simulink model "DC_Motor_Control_PM"  (R2022b)
settings: Solver=ode23s  StartTime=0.0  StopTime=0.2  RelTol=1e-3  EnableMultiTasking=on
values from neighbouring files (symbols this model uses):
  B = 0.01    [PI_design_DC_PM.m]
  J = 6e-5    (= 6e-05)    [PI_design_DC_PM.m]
  K = Ke    (= 0.04)    [PI_design_DC_PM.m]
  kb_curr = 1/tauGc    (= 300)    [PI_design_DC_PM.m]
  kb_speed = 1/tauGm    (= 166.666666667)    [PI_design_DC_PM.m]
  ki_curr = Ccurr.Ki    [PI_design_DC_PM.m]
  ki_speed = Cspeed.Ki    [PI_design_DC_PM.m]
  kp_curr = Ccurr.Kp    [PI_design_DC_PM.m]
  kp_speed = Cspeed.Kp    [PI_design_DC_PM.m]
  La = 0.002    [PI_design_DC_PM.m]
  Ra = 0.6    [PI_design_DC_PM.m]
libraries: slpidlib x2
settings Model: Creator=matti  LastModifiedBy=benve
settings SolverCC: AlgebraicLoopSolver=TrustRegion
settings DataIOCC: LimitDataPoints=on  SaveFormat=Array  ReturnWorkspaceOutputs=off
settings OptimizationCC: LifeSpan=inf
settings DebuggingCC: SolverPrmCheckMsg=warning  UnconnectedInputMsg=warning  UnconnectedOutputMsg=warning  UnconnectedLineMsg=warning  SFUnexpectedBacktrackingDiag=warning  SFNoUnconditionalDefaultTransitionDiag=warning  SFExecutionAtInitializationDiag=none  SFMachineParentedDataDiag=warning  ArithmeticOperatorsInVariantConditions=warning
settings HardwareCC: ProdBitPerPointer=32  ProdBitPerSizeT=32  ProdBitPerPtrDiffT=32  ProdLargestAtomicFloat=None  ProdIntDivRoundTo=Undefined  ProdEndianess=Unspecified  ProdWordSize=32  ProdHWDeviceType=32-bit Generic
settings ModelReferenceCC: EnableRefExpFcnMdlSchedulingChecks=on  PropagateSignalLabelsOutOfModel=off
settings SFSimCC: SimUseLocalCustomCode=off  CustomCodeUndefinedFunction=UseInterfaceOnly
settings RTWCC: RTWUseLocalCustomCode=off
settings CodeAppCC: StateflowObjectComments=on
settings GRTTargetCC: TargetLangStandard=C89/C90 (ANSI)
settings ConfigComp: CovMetricSettings=dw  CovSaveCumulativeToWorkspaceVar=on  CovSaveSingleToWorkspaceVar=on  CovExternalEMLEnable=off  CovSFcnEnable=off

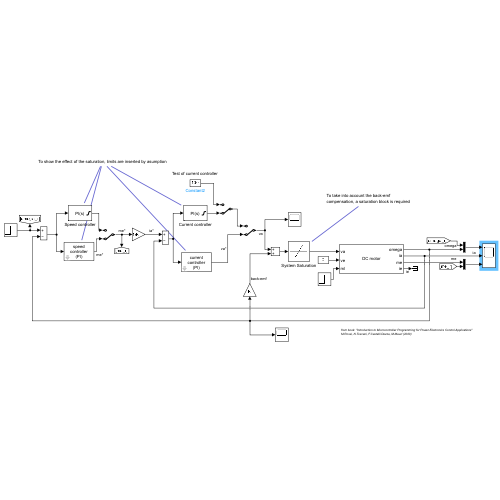
[thumbnail: Simulink's stored preview of the top-level diagram]
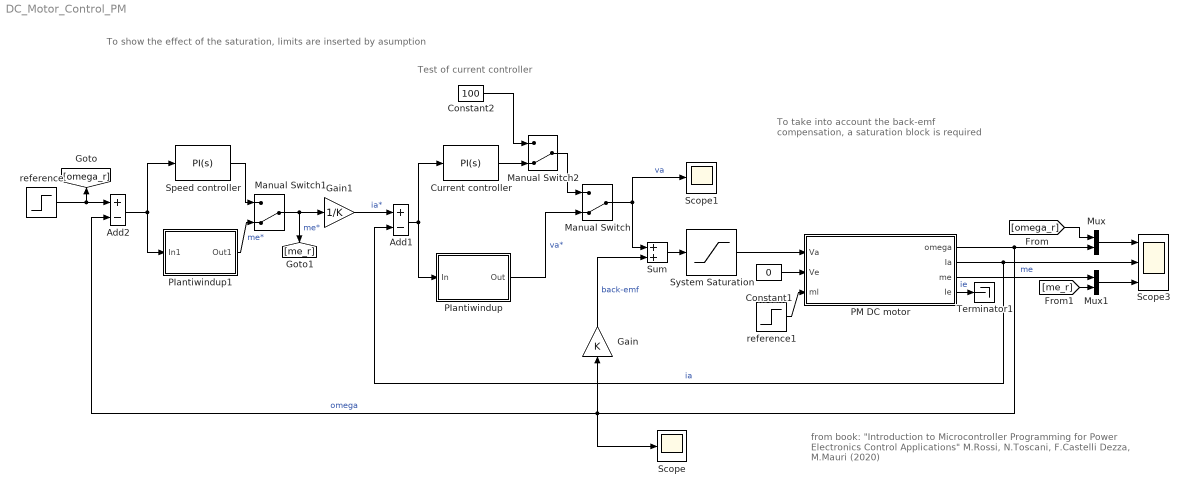
== system DC_Motor_Control_PM ==
  note: To take into account the back-emf
      | compensation, a saturation block is required
  note: To show the effect of the saturation, limits are inserted by asumption
  note: Test of current controller
  note: from book: "Introduction to Microcontroller Programming for Power Electronics Control Applications"
      | M.Rossi, N.Toscani, F.Castelli Dezza, M.Mauri (2020)
  Add1 : Sum  Inputs=+-
  Add2 : Sum  Inputs=+-
  Constant1 : Constant  Value=0
  Constant2 : Constant  Value=100
  Current controller : slpidlib/PID Controller  Controller=PI  Form=Parallel  TimeDomain=Continuous-time  UseExternalTs=off  SampleTime=-1  IntegratorMethod=Forward Euler  FilterMethod=Forward Euler  ControllerParametersSource=internal  P=kp_curr  I=ki_curr  UseKiTs=off  D=0  N=100  UseFilter=on  TunerSelectOption=Transfer Function Based (PID Tuner App)  InitialConditionSource=internal  InitialConditionForIntegrator=0  InitialConditionForFilter=0  DifferentiatorICPrevScaledInput=0  ExternalReset=none  TrackingMode=off  Kt=1  LimitOutput=on  SatLimitsSource=internal  UpperSaturationLimit=600*1.5  LowerSaturationLimit=-600*1.5  LinearizeAsGain=on  AntiWindupMode=back-calculation  Kb=kb_curr  LimitIntegrator=off  UpperIntegratorSaturationLimit=inf  LowerIntegratorSaturationLimit=-inf  POutMin=[]  POutMax=[]  IOutMin=[]  IOutMax=[]  DOutMin=[]  DOutMax=[]  NOutMin=[]  NOutMax=[]  SumOutMin=[]  SumOutMax=[]  SaturationOutMin=[]  SaturationOutMax=[]  PParamMin=[]  PParamMax=[]  IParamMin=[]  IParamMax=[]  DParamMin=[]  DParamMax=[]  NParamMin=[]  NParamMax=[]  KbParamMin=[]  KbParamMax=[]  KtParamMin=[]  KtParamMax=[]  KbOutMin=[]  KbOutMax=[]  KtOutMin=[]  KtOutMax=[]  IntegratorOutMin=[]  IntegratorOutMax=[]  FilterOutMin=[]  FilterOutMax=[]  SumI1OutMin=[]  SumI1OutMax=[]  SumI2OutMin=[]  SumI2OutMax=[]  SumI3OutMin=[]  SumI3OutMax=[]  SumI4OutMin=[]  SumI4OutMax=[]  SumDOutMin=[]  SumDOutMax=[]  DifferentiatorOutMin=[]  DifferentiatorOutMax=[]  FilterDiffOutCoefMin=[]  FilterDiffOutCoefMax=[]  ReciprocalOutMin=[]  ReciprocalOutMax=[]  SumDenOutMin=[]  SumDenOutMax=[]  SumNumOutMin=[]  SumNumOutMax=[]  DivideOutMin=[]  DivideOutMax=[]  UdiffTsProdOutMin=[]  UdiffTsProdOutMax=[]  NTsProdOutMin=[]  NTsProdOutMax=[]  UintegralTsProdOutMin=[]  UintegralTsProdOutMax=[]  UngainTsProdOutMin=[]  UngainTsProdOutMax=[]  ClampingZeroOutDataTypeStr=Inherit: Inherit via back propagation  ClampingZeroOutMin=[]  ClampingZeroOutMax=[]  FilterDenConstantOutDataTypeStr=Inherit: Inherit via back propagation  FilterDenConstantOutMin=[]  FilterDenConstantOutMax=[]  PCopyOutDataTypeStr=Inherit: Inherit via back propagation  PCopyOutMin=[]  PCopyOutMax=[]  NCopyOutDataTypeStr=Inherit: Inherit via back propagation  NCopyOutMin=[]  NCopyOutMax=[]  IntegratorContinuousStateAttributes=''  IntegratorStateMustResolveToSignalObject=off  IntegratorRTWStateStorageClass=Auto  FilterContinuousStateAttributes=''  FilterStateMustResolveToSignalObject=off  FilterRTWStateStorageClass=Auto  ParallelPVariant=InternalParameters  IdealPVariant=Disabled  IVariant=InternalParameters  DVariant=Disabled  IntegratorVariant=Continuous  SatVariant=Enabled  AWVariant=BackCalculation  PCopyVariant=Disabled  TRVariant=Disabled  FdbkBlocksVariant=Forward  IdealPFdbkVariant=Disabled  SatFdbkVariant=Disabled  DerivativeFilterVariant=Disabled  NVariant=Disabled  NCopyVariant=Disabled_SignalSpec  FilterICVariant=Disabled  IntegratorICVariant=InternalICs  ExternalResetVariant=Disabled  TRSumVariant=Passthrough  SumFdbkVariant=Disabled  SumVariant=Sum_PI  TsampFilterVariant=InternalTs  TsampNgainVariant=Passthrough  TsampIntegralVariant=Passthrough  ExternalSaturationOutDataTypeStr=Inherit: Same as second input
  Gain : Gain  Gain=K
  Gain1 : Gain  Gain=1/K
  Manual Switch : ManualSwitch  CurrentSetting=0
  Manual Switch1 : ManualSwitch  CurrentSetting=0
  Manual Switch2 : ManualSwitch  CurrentSetting=0
  Mux : Mux  Inputs=2
  Mux1 : Mux  Inputs=2
  PIantiwindup : Subsystem  mask{Kp=kp_curr, Ki=ki_curr, sat_up=600, sat_down=-600}
      mask prompts: sat_up "Upper sat. limit"; sat_down "Lower Sat. Limit"
      mask Display: disp('current\ncontroller\n(PI)')
  PIantiwindup1 : Subsystem  mask{Kp=kp_speed, Ki=ki_speed, sat_up=1000, sat_down=-1000}
      mask prompts: sat_up "Upper sat. limit"; sat_down "Lower Sat. Limit"
      mask Display: disp('speed\ncontroller\n(PI)')
  PM DC motor : Subsystem
      mask Display:
      | disp('DC motor')
      | port_label('input', 1, 'va')
      | port_label('input', 2, 've')
      | port_label('input', 3, 'ml')
      | port_label('output', 1, 'omega')
      | port_label('output', 2, 'ia')
      | port_label('output', 3, 'me')
      | port_label('output', 4, 'ie')
  Scope : Scope
  Scope1 : Scope
  Scope3 : Scope  NumInputPorts=3
  Speed controller : slpidlib/PID Controller  Controller=PI  Form=Parallel  TimeDomain=Continuous-time  UseExternalTs=off  SampleTime=-1  IntegratorMethod=Forward Euler  FilterMethod=Forward Euler  ControllerParametersSource=internal  P=kp_speed  I=ki_speed  UseKiTs=off  D=0  N=100  UseFilter=on  TunerSelectOption=Transfer Function Based (PID Tuner App)  InitialConditionSource=internal  InitialConditionForIntegrator=0  InitialConditionForFilter=0  DifferentiatorICPrevScaledInput=0  ExternalReset=none  TrackingMode=off  Kt=1  LimitOutput=on  SatLimitsSource=internal  UpperSaturationLimit=1000  LowerSaturationLimit=-1000  LinearizeAsGain=on  AntiWindupMode=back-calculation  Kb=kb_speed  LimitIntegrator=off  UpperIntegratorSaturationLimit=inf  LowerIntegratorSaturationLimit=-inf  POutMin=[]  POutMax=[]  IOutMin=[]  IOutMax=[]  DOutMin=[]  DOutMax=[]  NOutMin=[]  NOutMax=[]  SumOutMin=[]  SumOutMax=[]  SaturationOutMin=[]  SaturationOutMax=[]  PParamMin=[]  PParamMax=[]  IParamMin=[]  IParamMax=[]  DParamMin=[]  DParamMax=[]  NParamMin=[]  NParamMax=[]  KbParamMin=[]  KbParamMax=[]  KtParamMin=[]  KtParamMax=[]  KbOutMin=[]  KbOutMax=[]  KtOutMin=[]  KtOutMax=[]  IntegratorOutMin=[]  IntegratorOutMax=[]  FilterOutMin=[]  FilterOutMax=[]  SumI1OutMin=[]  SumI1OutMax=[]  SumI2OutMin=[]  SumI2OutMax=[]  SumI3OutMin=[]  SumI3OutMax=[]  SumI4OutMin=[]  SumI4OutMax=[]  SumDOutMin=[]  SumDOutMax=[]  DifferentiatorOutMin=[]  DifferentiatorOutMax=[]  FilterDiffOutCoefMin=[]  FilterDiffOutCoefMax=[]  ReciprocalOutMin=[]  ReciprocalOutMax=[]  SumDenOutMin=[]  SumDenOutMax=[]  SumNumOutMin=[]  SumNumOutMax=[]  DivideOutMin=[]  DivideOutMax=[]  UdiffTsProdOutMin=[]  UdiffTsProdOutMax=[]  NTsProdOutMin=[]  NTsProdOutMax=[]  UintegralTsProdOutMin=[]  UintegralTsProdOutMax=[]  UngainTsProdOutMin=[]  UngainTsProdOutMax=[]  ClampingZeroOutDataTypeStr=Inherit: Inherit via back propagation  ClampingZeroOutMin=[]  ClampingZeroOutMax=[]  FilterDenConstantOutDataTypeStr=Inherit: Inherit via back propagation  FilterDenConstantOutMin=[]  FilterDenConstantOutMax=[]  PCopyOutDataTypeStr=Inherit: Inherit via back propagation  PCopyOutMin=[]  PCopyOutMax=[]  NCopyOutDataTypeStr=Inherit: Inherit via back propagation  NCopyOutMin=[]  NCopyOutMax=[]  IntegratorContinuousStateAttributes=''  IntegratorStateMustResolveToSignalObject=off  IntegratorRTWStateStorageClass=Auto  FilterContinuousStateAttributes=''  FilterStateMustResolveToSignalObject=off  FilterRTWStateStorageClass=Auto  ParallelPVariant=InternalParameters  IdealPVariant=Disabled  IVariant=InternalParameters  DVariant=Disabled  IntegratorVariant=Continuous  SatVariant=Enabled  AWVariant=BackCalculation  PCopyVariant=Disabled  TRVariant=Disabled  FdbkBlocksVariant=Forward  IdealPFdbkVariant=Disabled  SatFdbkVariant=Disabled  DerivativeFilterVariant=Disabled  NVariant=Disabled  NCopyVariant=Disabled_SignalSpec  FilterICVariant=Disabled  IntegratorICVariant=InternalICs  ExternalResetVariant=Disabled  TRSumVariant=Passthrough  SumFdbkVariant=Disabled  SumVariant=Sum_PI  TsampFilterVariant=InternalTs  TsampNgainVariant=Passthrough  TsampIntegralVariant=Passthrough  ExternalSaturationOutDataTypeStr=Inherit: Same as second input
  Sum : Sum
  System Saturation : Saturate  UpperLimit=600  LowerLimit=-600
  Terminator1 : Terminator
  reference : Step  Time=0.05  After=300  SampleTime=0
  reference1 : Step  Time=0.05  After=3  SampleTime=0
  wires:
  PM DC motor/1(omega) -> Gain/1, Add2/2, Scope/1, Mux/2  "omega"
  PIantiwindup/1(Out) -> Manual Switch/2  "va*"
  Manual Switch/1 -> Sum/1, Scope1/1  "va"
  reference1/1 -> PM DC motor/3(ml)
  Constant1/1 -> PM DC motor/2(Ve)
  Add1/1 -> PIantiwindup/1(In), Current controller/1
  Manual Switch1/1 -> [me_r], Gain1/1  "me*"
  reference/1 -> Add2/1, [omega_r]
  PM DC motor/2(Ia) -> Add1/2, Scope3/2  "ia"
  PM DC motor/3(me) -> Mux1/1  "me"
  Gain1/1 -> Add1/1  "ia*"
  Mux/1 -> Scope3/1
  [me_r] -> Mux1/2
  Mux1/1 -> Scope3/3
  [omega_r] -> Mux/1
  PM DC motor/4(Ie) -> Terminator1/1  "ie"
  PIantiwindup1/1(Out1) -> Manual Switch1/2  "me*"
  Speed controller/1 -> Manual Switch1/1
  Add2/1 -> Speed controller/1, PIantiwindup1/1(In1)
  Current controller/1 -> Manual Switch2/2
  Constant2/1 -> Manual Switch2/1
  Manual Switch2/1 -> Manual Switch/1
  System Saturation/1 -> PM DC motor/1(Va)
  Sum/1 -> System Saturation/1
  Gain/1 -> Sum/2  "back-emf"

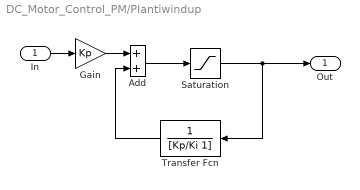
== system DC_Motor_Control_PM/PIantiwindup ==
  In : Inport
  Add : Sum
  Gain : Gain  Gain=Kp
  Saturation : Saturate  UpperLimit=sat_up  LowerLimit=sat_down
  Transfer Fcn : TransferFcn  Denominator=[Kp/Ki 1]
  Out : Outport  VectorParamsAs1DForOutWhenUnconnected=off
  wires:
  Saturation/1 -> Out/1, Transfer Fcn/1
  In/1 -> Gain/1
  Gain/1 -> Add/1
  Transfer Fcn/1 -> Add/2
  Add/1 -> Saturation/1

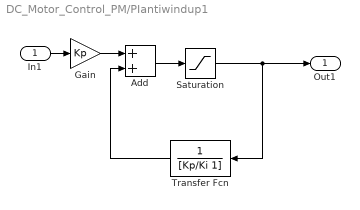
== system DC_Motor_Control_PM/PIantiwindup1 ==
  In1 : Inport
  Add : Sum
  Gain : Gain  Gain=Kp
  Saturation : Saturate  UpperLimit=sat_up  LowerLimit=sat_down
  Transfer Fcn : TransferFcn  Denominator=[Kp/Ki 1]
  Out1 : Outport  VectorParamsAs1DForOutWhenUnconnected=off
  wires:
  Transfer Fcn/1 -> Add/2
  Add/1 -> Saturation/1
  Gain/1 -> Add/1
  In1/1 -> Gain/1
  Saturation/1 -> Transfer Fcn/1, Out1/1

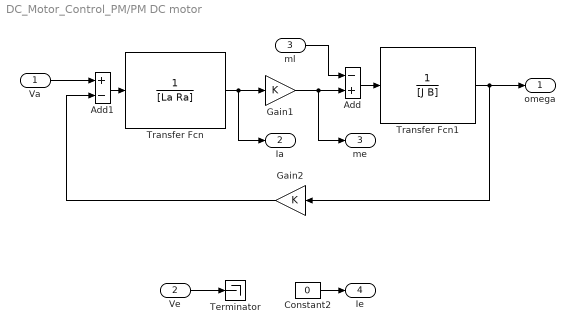
== system DC_Motor_Control_PM/PM DC motor ==
  Va : Inport
  Ve : Inport  Port=2
  ml : Inport  Port=3
  Add : Sum  Inputs=-+
  Add1 : Sum  Inputs=+-
  Constant2 : Constant  Value=0
  Gain1 : Gain  Gain=K
  Gain2 : Gain  Gain=K
  Terminator : Terminator
  Transfer Fcn : TransferFcn  Denominator=[La Ra]
  Transfer Fcn1 : TransferFcn  Denominator=[J B]
  omega : Outport  VectorParamsAs1DForOutWhenUnconnected=off
  Ia : Outport  Port=2  VectorParamsAs1DForOutWhenUnconnected=off
  me : Outport  Port=3  VectorParamsAs1DForOutWhenUnconnected=off
  Ie : Outport  Port=4  VectorParamsAs1DForOutWhenUnconnected=off
  wires:
  ml/1 -> Add/1
  Add/1 -> Transfer Fcn1/1
  Add1/1 -> Transfer Fcn/1
  Transfer Fcn/1 -> Ia/1, Gain1/1
  Gain1/1 -> Add/2, me/1
  Va/1 -> Add1/1
  Transfer Fcn1/1 -> omega/1, Gain2/1
  Gain2/1 -> Add1/2
  Ve/1 -> Terminator/1
  Constant2/1 -> Ie/1
